simulink model "tank_PP"  (R2021b)
settings: Solver=VariableStepAuto  StartTime=0.0  StopTime=5  RelTol=1e-3
undefined symbols (not defined in the file): A, b, Be, Bh, Bm, Bs, C, Continuous, d, Dh, Fc, Flp, forceVariance, Jh, Ke, Km, Ks, Mm, Ms, Ph, posVariance, R, Time, Ts, xe
libraries: ctrlSharedLib x2
settings Model: Creator=buse  LastModifiedBy=buse

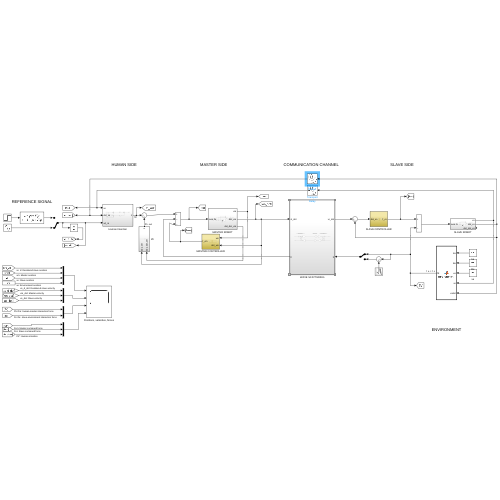
[thumbnail: Simulink's stored preview of the top-level diagram]
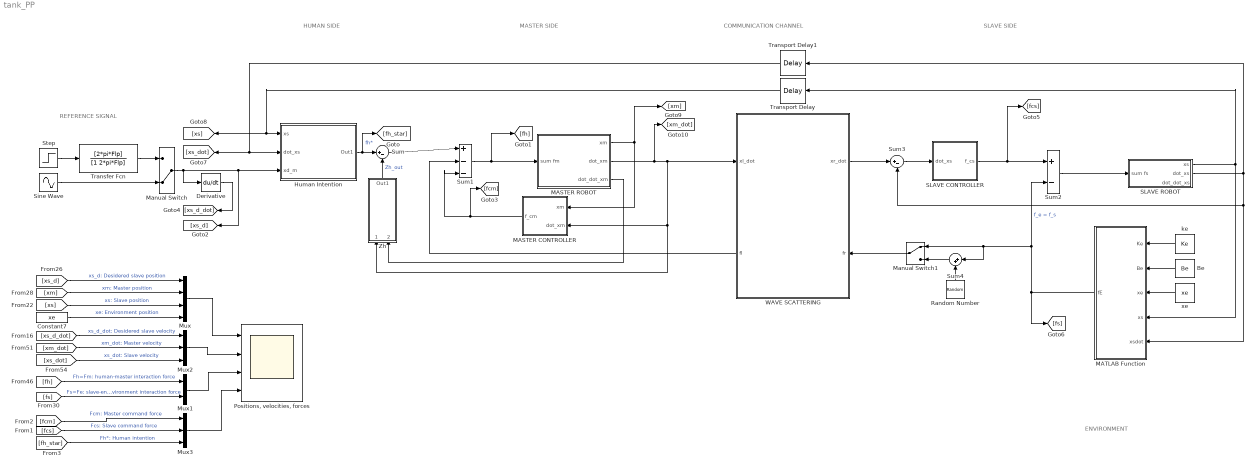
== system tank_PP ==
  note: SLAVE SIDE
  note: COMMUNICATION CHANNEL
  note: MASTER SIDE
  note: REFERENCE SIGNAL
  note: ENVIRONMENT
  note: HUMAN SIDE
  Be : Constant  Value=Be
  Constant7 : Constant  Value=xe
  Derivative : Derivative
  Human Intention : Subsystem
  MASTER CONTROLLER : Subsystem
  MASTER ROBOT : Subsystem
  MATLAB Function : MATLAB Function  TreatAsAtomicUnit=on
  Manual Switch : ManualSwitch  CurrentSetting=0
  Manual Switch1 : ManualSwitch
  Mux : Mux
  Mux1 : Mux  Inputs=2
  Mux2 : Mux  Inputs=3
  Mux3 : Mux  Inputs=3
  "Positions, velocities, forces" : Scope  NumInputPorts=4
  Random Number : RandomNumber  Variance=forceVariance  SampleTime=Ts
  SLAVE CONTROLLER : Subsystem
  SLAVE ROBOT : Subsystem
  Sine Wave : Sin  Amplitude=A  Frequency=Fc*2*pi  SampleTime=0
  Step : Step  After=A  SampleTime=0
  Sum : Sum  Inputs=|+-
  Sum1 : Sum  Inputs=+--
  Sum2 : Sum  Inputs=+-
  Sum3 : Sum  Inputs=|+-
  Sum4 : Sum  Inputs=|++
  Transfer Fcn : TransferFcn  Numerator=[2*pi*Flp]  Denominator=[1 2*pi*Flp]
  Transport Delay : TransportDelay  DelayTime=d
  Transport Delay1 : TransportDelay  DelayTime=d
  WAVE SCATTERING : Subsystem
      settings: PortSchema="{\"entries\":[{\"content\":{\"sides\":[{\"content\":{\"connectorIds\":[\"In1\",\"Out2\"]},\"type\":\"ConnectorPlacement.EquallySpacedRectSide\",\"uuid\":\"48d02bf4-4cb9-4160-ab12-3229c46703a5\"},{\"content\":{\"connectorIds\":[\"Out1\",\"In2\"],\"side\":\"RIGHT\"},\"type\":\"ConnectorPlacement.EquallySpacedRectSide\",\"uuid\":\"ea81abd4-a31d-438b-9926-fe0cbf939221\"},{\"content\":{\"connectorIds\":[],\"side\":\"TOP\"},\"type\":\"ConnectorPlacement.EquallySpacedRectSide\",\"uuid\":\"1e510e84-16ab-408c-8c2c-25a01bc4c05a\"}]},\"type\":\"ConnectorPlacement.EquallySpacedConnector\",\"uuid\":\"0e85e32e-1f39-4fe2-85f3-40fbe1858f78\"}],\"packageUris\":[\"http://schema.mathworks.com/mf0/Connector/R2020b\"],\"version\":\"1.0\"}"
  Zh : Subsystem
  ke : Constant  Value=Ke
  xe : Constant  Value=xe
  wires:
  [fcs] -> Mux3/2  "Fcs: Slave command force"
  [xm] -> Mux/2  "xm: Master position"
  Zh/1(Out1) -> Sum/2  "Zh_out"
  MASTER ROBOT/3(dot_dot_xm) -> Zh/2(dot_dot_xm)
  Sine Wave/1 -> Manual Switch/2
  [xm_dot] -> Mux2/2  "xm_dot: Master velocity"
  Mux1/1 -> "Positions, velocities, forces"/3
  Mux/1 -> "Positions, velocities, forces"/1
  ke/1 -> MATLAB Function/1(Ke)
  xe/1 -> MATLAB Function/3(xe)
  [xs_d] -> Mux/1  "xs_d: Desidered slave position"
  MASTER ROBOT/1(xm) -> [xm], MASTER CONTROLLER/1(xm)
  Sum/1 -> Sum1/1
  Step/1 -> Transfer Fcn/1
  SLAVE ROBOT/1(xs) -> Transport Delay/1, MATLAB Function/4(xs)
  [fcm] -> Mux3/1  "Fcm: Master command force"
  Transfer Fcn/1 -> Manual Switch/1
  [fh_star] -> Mux3/3  "Fh*: Human intention"
  Mux2/1 -> "Positions, velocities, forces"/2
  Derivative/1 -> [xs_d_dot]
  [xs_d_dot] -> Mux2/1  "xs_d_dot: Desidered slave velocity"
  [fh] -> Mux1/1  "Fh=Fm: human-master interaction force"
  [fs] -> Mux1/2  "Fs=Fe: slave-environment interaction force"
  SLAVE CONTROLLER/1(f_cs) -> [fcs], Sum2/1
  Be/1 -> MATLAB Function/2(Be)
  [xs] -> Mux/3  "xs: Slave position"
  MASTER ROBOT/2(dot_xm) -> [xm_dot], Zh/1(dot_xm), MASTER CONTROLLER/2(dot_xm), WAVE SCATTERING/1(xl_dot)
  Sum1/1 -> [fh], MASTER ROBOT/1(sum fm)
  MATLAB Function/1(fE) -> Manual Switch1/1, Sum4/1, Sum2/2, [fs]  "f_e = f_s"
  MASTER CONTROLLER/1(f_cm) -> Sum1/3, [fcm]
  Human Intention/1(Out1) -> [fh_star], Sum/1  "fh*"
  SLAVE ROBOT/2(dot_xs) -> Transport Delay1/1, Sum3/2, MATLAB Function/5(xsdot)
  Manual Switch/1 -> Derivative/1, Human Intention/3(xd_m), [xs_d]
  Sum2/1 -> SLAVE ROBOT/1(sum fs)
  [xs_dot] -> Mux2/3  "xs_dot: Slave velocity"
  Mux3/1 -> "Positions, velocities, forces"/4
  Constant7/1 -> Mux/4  "xe: Environment position"
  Sum3/1 -> SLAVE CONTROLLER/1(dot_xs)
  WAVE SCATTERING/1(xr_dot) -> Sum3/1
  WAVE SCATTERING/2(fl) -> Sum1/2
  Manual Switch1/1 -> WAVE SCATTERING/2(fr)
  Sum4/1 -> Manual Switch1/2
  Random Number/1 -> Sum4/2
  Transport Delay/1 -> Human Intention/1(xs), [xs]
  Transport Delay1/1 -> [xs_dot], Human Intention/2(dot_xs)

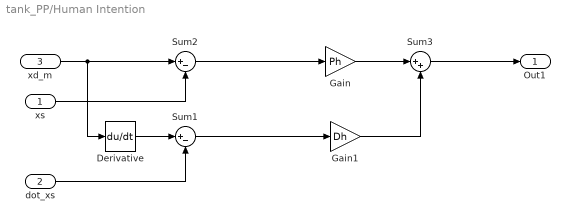
== system tank_PP/Human Intention ==
  xs : Inport
  dot_xs : Inport  Port=2
  xd_m : Inport  Port=3
  Derivative : Derivative
  Gain : Gain  Gain=Ph
  Gain1 : Gain  Gain=Dh
  Sum1 : Sum  Inputs=|+-
  Sum2 : Sum  Inputs=|+-
  Sum3 : Sum  Inputs=|++
  Out1 : Outport
  wires:
  xs/1 -> Sum2/2
  dot_xs/1 -> Sum1/2
  Sum2/1 -> Gain/1
  Sum1/1 -> Gain1/1
  Gain1/1 -> Sum3/2
  Gain/1 -> Sum3/1
  Sum3/1 -> Out1/1
  xd_m/1 -> Derivative/1, Sum2/1
  Derivative/1 -> Sum1/1

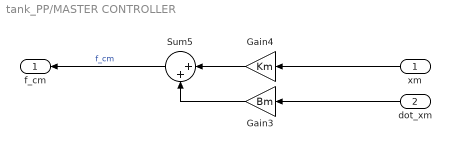
== system tank_PP/MASTER CONTROLLER ==
  xm : Inport
  dot_xm : Inport  Port=2
  Gain3 : Gain  Gain=Bm
  Gain4 : Gain  Gain=Km
  Sum5 : Sum  Inputs=|++
  f_cm : Outport
  wires:
  Gain4/1 -> Sum5/1
  Gain3/1 -> Sum5/2
  dot_xm/1 -> Gain3/1
  Sum5/1 -> f_cm/1  "f_cm"
  xm/1 -> Gain4/1

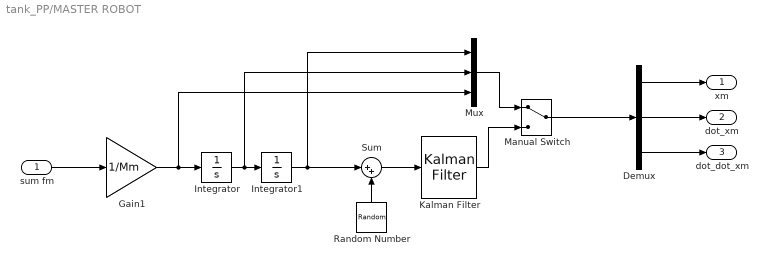
== system tank_PP/MASTER ROBOT ==
  sum fm : Inport
  Demux : Demux  Outputs=3
  Gain1 : Gain  Gain=1/Mm
  Integrator : Integrator
  Integrator1 : Integrator
  Kalman Filter : ctrlSharedLib/Kalman Filter  TimeDomain=Continuous-Time  UseCurrentEstimator=on  ModelSource=Individual A, B, C, D matrices  ModelSourceVariable=ss(0.95,1,1,0,1)  A=A  B=1  C=C  D=0  NumberOfStates=1  NumberOfInputs=1  NumberOfOutputs=1  InitialEstimateSource=Dialog  X0=0  P0=10  UseK=off  UseGH=off  NumberOfProcessNoiseInputs=1  G=1  TimeInvariantG=on  H=0  TimeInvariantH=on  Q=Q  TimeInvariantQ=on  R=R  TimeInvariantR=on  N=0  TimeInvariantN=on  AddInputPort=off  AddEnablePort=off  OutputEstimatedY=off  OutputP=off  Ts=-1
  Manual Switch : ManualSwitch
  Mux : Mux  Inputs=3
  Random Number : RandomNumber  Variance=posVariance  SampleTime=Ts
  Sum : Sum  Inputs=|++
  xm : Outport
  dot_xm : Outport  Port=2
  dot_dot_xm : Outport  Port=3
  wires:
  sum fm/1 -> Gain1/1
  Gain1/1 -> Mux/3, Integrator/1
  Integrator1/1 -> Mux/1, Sum/1
  Integrator/1 -> Mux/2, Integrator1/1
  Random Number/1 -> Sum/2
  Sum/1 -> Kalman Filter/1
  Mux/1 -> Manual Switch/1
  Kalman Filter/1 -> Manual Switch/2
  Manual Switch/1 -> Demux/1
  Demux/1 -> xm/1
  Demux/2 -> dot_xm/1
  Demux/3 -> dot_dot_xm/1

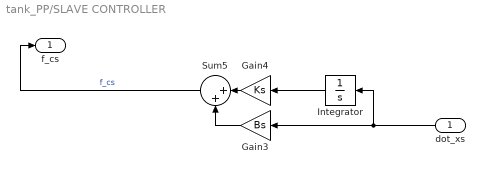
== system tank_PP/SLAVE CONTROLLER ==
  dot_xs : Inport
  Gain3 : Gain  Gain=Bs
  Gain4 : Gain  Gain=Ks
  Integrator : Integrator
  Sum5 : Sum  Inputs=|++
  f_cs : Outport
  wires:
  Gain4/1 -> Sum5/1
  Gain3/1 -> Sum5/2
  Sum5/1 -> f_cs/1  "f_cs"
  Integrator/1 -> Gain4/1
  dot_xs/1 -> Integrator/1, Gain3/1

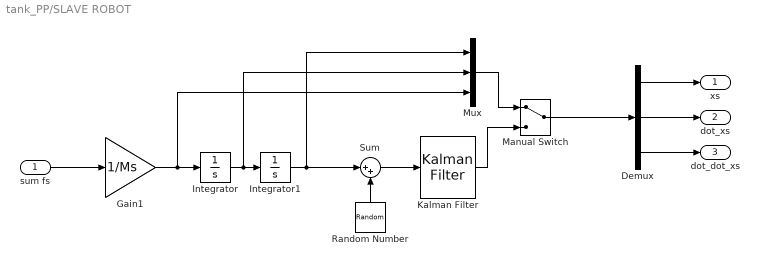
== system tank_PP/SLAVE ROBOT ==
  sum fs : Inport
  Demux : Demux  Outputs=3
  Gain1 : Gain  Gain=1/Ms
  Integrator : Integrator
  Integrator1 : Integrator
  Kalman Filter : ctrlSharedLib/Kalman Filter  TimeDomain=Continuous-Time  UseCurrentEstimator=on  ModelSource=Individual A, B, C, D matrices  ModelSourceVariable=ss(0.95,1,1,0,1)  A=A  B=1  C=C  D=0  NumberOfStates=1  NumberOfInputs=1  NumberOfOutputs=1  InitialEstimateSource=Dialog  X0=0  P0=10  UseK=off  UseGH=off  NumberOfProcessNoiseInputs=1  G=1  TimeInvariantG=on  H=0  TimeInvariantH=on  Q=Q  TimeInvariantQ=on  R=R  TimeInvariantR=on  N=0  TimeInvariantN=on  AddInputPort=off  AddEnablePort=off  OutputEstimatedY=off  OutputP=off  Ts=-1
  Manual Switch : ManualSwitch
  Mux : Mux  Inputs=3
  Random Number : RandomNumber  Variance=posVariance  SampleTime=Ts
  Sum : Sum  Inputs=|++
  xs : Outport
  dot_xs : Outport  Port=2
  dot_dot_xs : Outport  Port=3
  wires:
  sum fs/1 -> Gain1/1
  Sum/1 -> Kalman Filter/1
  Demux/3 -> dot_dot_xs/1
  Demux/2 -> dot_xs/1
  Integrator/1 -> Mux/2, Integrator1/1
  Manual Switch/1 -> Demux/1
  Kalman Filter/1 -> Manual Switch/2
  Random Number/1 -> Sum/2
  Gain1/1 -> Mux/3, Integrator/1
  Mux/1 -> Manual Switch/1
  Demux/1 -> xs/1
  Integrator1/1 -> Mux/1, Sum/1

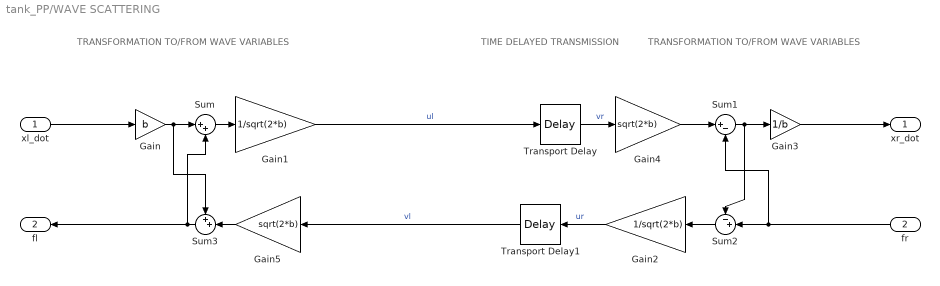
== system tank_PP/WAVE SCATTERING ==
  note: TIME DELAYED
      | TRANSMISSION
  note: TRANSFORMATION TO/FROM
      | WAVE VARIABLES
  note: TRANSFORMATION TO/FROM
      | WAVE VARIABLES
  xl_dot : Inport
  fr : Inport  Port=2
  Gain : Gain  Gain=b
  Gain1 : Gain  Gain=1/sqrt(2*b)
  Gain2 : Gain  Gain=1/sqrt(2*b)
  Gain3 : Gain  Gain=1/b
  Gain4 : Gain  Gain=sqrt(2*b)
  Gain5 : Gain  Gain=sqrt(2*b)
  Sum : Sum  Inputs=|++
  Sum1 : Sum  Inputs=|+-
  Sum2 : Sum  Inputs=-+|
  Sum3 : Sum  Inputs=++|
  Transport Delay : TransportDelay  DelayTime=d
  Transport Delay1 : TransportDelay  DelayTime=d
  xr_dot : Outport
  fl : Outport  Port=2
  wires:
  Gain/1 -> Sum3/1, Sum/1
  Sum/1 -> Gain1/1
  Gain4/1 -> Sum1/1
  Sum1/1 -> Sum2/1, Gain3/1
  Sum2/1 -> Gain2/1
  Gain5/1 -> Sum3/2
  Sum3/1 -> fl/1, Sum/2
  Gain1/1 -> Transport Delay/1  "ul"
  Transport Delay/1 -> Gain4/1  "vr"
  Gain2/1 -> Transport Delay1/1  "ur"
  Transport Delay1/1 -> Gain5/1  "vl"
  xl_dot/1 -> Gain/1
  Gain3/1 -> xr_dot/1
  fr/1 -> Sum1/2, Sum2/2

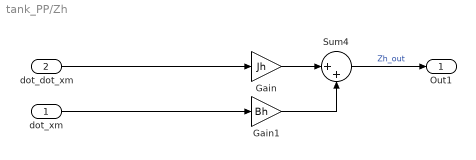
== system tank_PP/Zh ==
  dot_xm : Inport
  dot_dot_xm : Inport  Port=2
  Gain : Gain  Gain=Jh
  Gain1 : Gain  Gain=Bh
  Sum4 : Sum  Inputs=|++
  Out1 : Outport
  wires:
  dot_dot_xm/1 -> Gain/1
  Gain1/1 -> Sum4/2
  Gain/1 -> Sum4/1
  Sum4/1 -> Out1/1  "Zh_out"
  dot_xm/1 -> Gain1/1

== matlab function tank_PP/MATLAB Function ==
  data: Ke input; fE output; Be input; xe input; xs input; xsdot input
function fE = environment(Ke, Be, xe, xs, xsdot)
    if xs > xe
        fE = Ke * (xs - xe) + Be * xsdot; % Plot both contributions Ke and Be
    else
        fE = 0;
    end
end
